simulink model "Three_phase"  (R2015a)
settings: Solver=ode45  StartTime=0.0  StopTime=10.0  RelTol=1e-3
undefined symbols (not defined in the file): Vdc
libraries: simulink x21
settings Model: Creator=Caner  LastModifiedBy=Caner

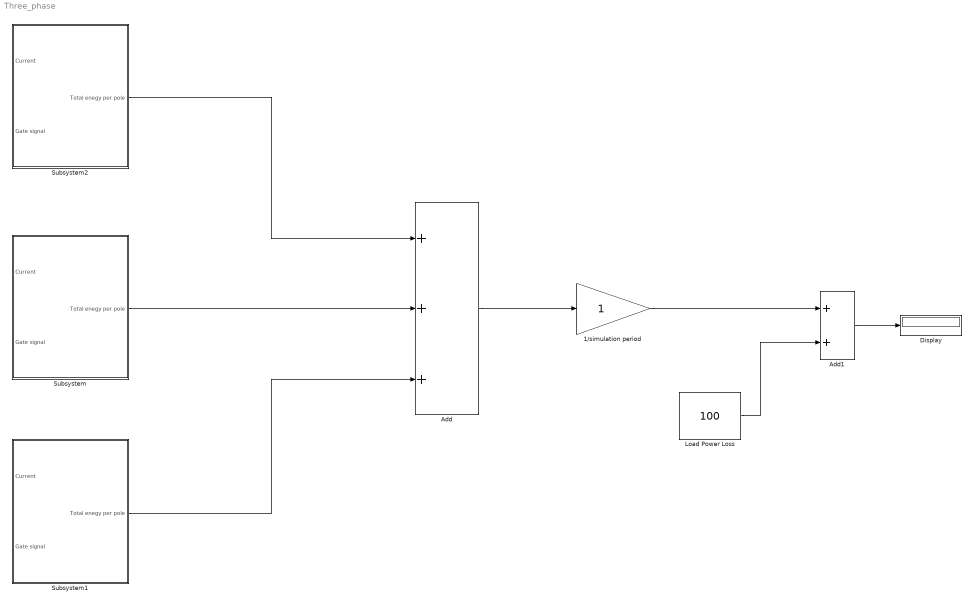
== system Three_phase ==
  1/simulation period : Gain
  Add : Sum  Inputs=+++
  Add1 : Sum
  Display : Display
  Load Power Loss : Constant  Value=100
  Subsystem : Subsystem
  Subsystem1 : Subsystem
  Subsystem2 : Subsystem
  wires:
  Subsystem2/1(Total enegy per pole) -> Add/1
  Subsystem/1(Total enegy per pole) -> Add/2
  Subsystem1/1(Total enegy per pole) -> Add/3
  Add/1 -> 1/simulation period/1
  1/simulation period/1 -> Add1/1
  Load Power Loss/1 -> Add1/2
  Add1/1 -> Display/1

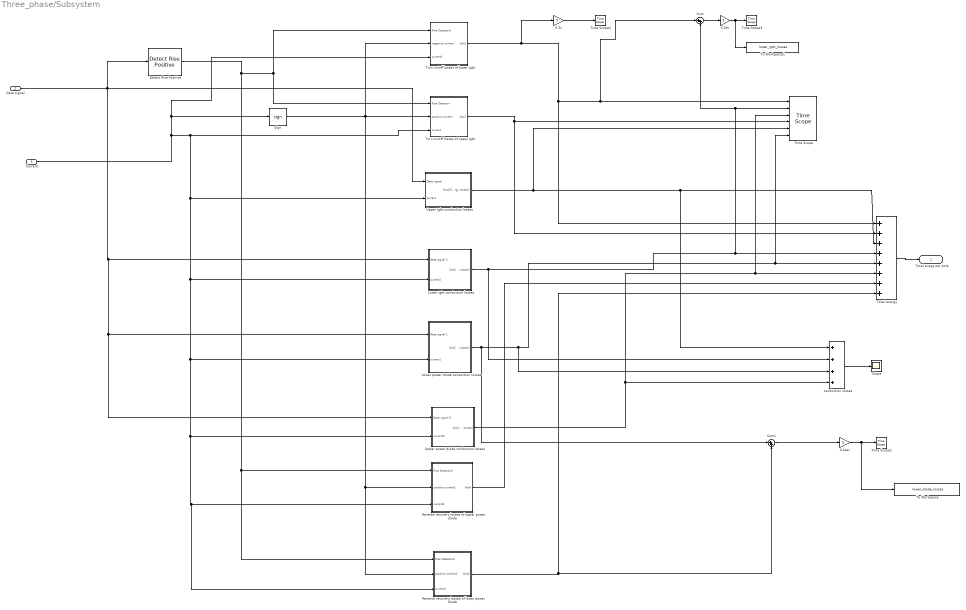
== system Three_phase/Subsystem ==
  Current : Inport
  "Gate signal " : Inport  Port=2
  0.2s : Gain  Gain=5
  0.2sec : Gain  Gain=5
  "0.2sn " : Gain  Gain=5
  Detect Rise Positive : simulink/Logic and Bit Operations/Detect Rise Positive  vinit=0  InputProcessing=Inherited  OutDataTypeStr=boolean
  Lower igbt conduction losses : Subsystem
  Lower power diode conduction losses : Subsystem
  "Reverse recovery losses of lower power diode " : Subsystem
  "Reverse recovery losses of upper power diode " : Subsystem
  Scope : Scope
      settings: SaveName=ScopeData3
  Sign : Signum
  Sum : Sum  Inputs=|++
  Sum1 : Sum  Inputs=|++
  Time Scope : TimeScope  DefaultConfigurationName=spbscopes.TimeScopeBlockCfg  NumInputPorts=6
  Time Scope1 : TimeScope  DefaultConfigurationName=spbscopes.TimeScopeBlockCfg
  Time Scope2 : TimeScope  DefaultConfigurationName=spbscopes.TimeScopeBlockCfg
  Time Scope3 : TimeScope  DefaultConfigurationName=spbscopes.TimeScopeBlockCfg
  To Workspace : ToWorkspace  VariableName=lower_diode_losses  SaveFormat=Timeseries  SampleTime=-1
  To Workspace1 : ToWorkspace  VariableName=lower_igbt_losses  SaveFormat=Timeseries  SampleTime=-1
  "Total energy " : Sum  Inputs=++++++++
  "Turn on/off losses of lower igbt " : Subsystem
  "Turn on/off losses of upper igbt " : Subsystem
  Upper igbt conduction losses : Subsystem
  Upper power diode conduction losses : Subsystem
  conduction losses : Sum  Inputs=++++
  Total enegy per pole : Outport
  wires:
  Current/1 -> Sign/1, "Turn on/off losses of lower igbt "/3(current1), "Turn on/off losses of upper igbt "/3(current), Upper igbt conduction losses/2(current), Lower igbt conduction losses/2(current2), Lower power diode conduction losses/2(current1), Upper power diode conduction losses/2(current3), "Reverse recovery losses of upper power diode "/3(current3), "Reverse recovery losses of lower power diode "/3(current2)
  Upper igbt conduction losses/1(Out1(Energy losses)) -> "Total energy "/3, conduction losses/1, Time Scope/5
  "Gate signal "/1 -> Detect Rise Positive/1, Upper igbt conduction losses/1("Gate signal "), Lower igbt conduction losses/1(Gate signal 2), Lower power diode conduction losses/1(Gate signal 1), Upper power diode conduction losses/1(Gate signal 3)
  Lower igbt conduction losses/1(Out3 (Energy losses)) -> "Total energy "/4, Sum/2, Time Scope/2, conduction losses/2
  "0.2sn "/1 -> Time Scope3/1, To Workspace1/1
  Detect Rise Positive/1 -> "Turn on/off losses of lower igbt "/1(Rise Detector1), "Turn on/off losses of upper igbt "/1(Rise Detector), "Reverse recovery losses of upper power diode "/1(Rise Detector3), "Reverse recovery losses of lower power diode "/1(Rise Detector2)
  Sum/1 -> "0.2sn "/1
  Upper power diode conduction losses/1(Out4 (Energy losses)) -> "Total energy "/6, Time Scope/3, conduction losses/4
  "Total energy "/1 -> Total enegy per pole/1
  0.2sec/1 -> Time Scope1/1, To Workspace/1
  Sum1/1 -> 0.2sec/1
  "Reverse recovery losses of upper power diode "/1(Out4) -> "Total energy "/7
  "Turn on/off losses of upper igbt "/1(Out1) -> Time Scope/4, "Total energy "/2
  conduction losses/1 -> Scope/1
  Sign/1 -> "Turn on/off losses of upper igbt "/2(positive current), "Turn on/off losses of lower igbt "/2(negative current), "Reverse recovery losses of lower power diode "/2(positive current1), "Reverse recovery losses of upper power diode "/2(positive current2)
  Lower power diode conduction losses/1(Out2 (Energy losses)) -> "Total energy "/5, Time Scope/6, conduction losses/3, Sum1/1
  0.2s/1 -> Time Scope2/1
  "Reverse recovery losses of lower power diode "/1(Out3) -> "Total energy "/8, Sum1/2
  "Turn on/off losses of lower igbt "/1(Out2) -> "Total energy "/1, Time Scope/1, Sum/1, 0.2s/1

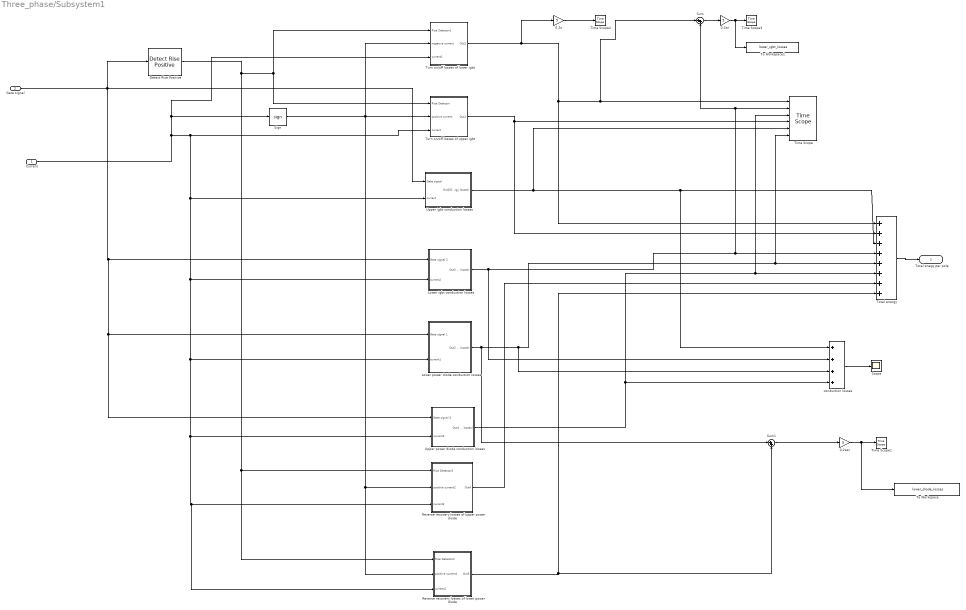
== system Three_phase/Subsystem1 ==
  Current : Inport
  "Gate signal " : Inport  Port=2
  0.2s : Gain  Gain=5
  0.2sec : Gain  Gain=5
  "0.2sn " : Gain  Gain=5
  Detect Rise Positive : simulink/Logic and Bit Operations/Detect Rise Positive  vinit=0  InputProcessing=Inherited  OutDataTypeStr=boolean
  Lower igbt conduction losses : Subsystem
  Lower power diode conduction losses : Subsystem
  "Reverse recovery losses of lower power diode " : Subsystem
  "Reverse recovery losses of upper power diode " : Subsystem
  Scope : Scope
      settings: SaveName=ScopeData3
  Sign : Signum
  Sum : Sum  Inputs=|++
  Sum1 : Sum  Inputs=|++
  Time Scope : TimeScope  DefaultConfigurationName=spbscopes.TimeScopeBlockCfg  NumInputPorts=6
  Time Scope1 : TimeScope  DefaultConfigurationName=spbscopes.TimeScopeBlockCfg
  Time Scope2 : TimeScope  DefaultConfigurationName=spbscopes.TimeScopeBlockCfg
  Time Scope3 : TimeScope  DefaultConfigurationName=spbscopes.TimeScopeBlockCfg
  To Workspace : ToWorkspace  VariableName=lower_diode_losses  SaveFormat=Timeseries  SampleTime=-1
  To Workspace1 : ToWorkspace  VariableName=lower_igbt_losses  SaveFormat=Timeseries  SampleTime=-1
  "Total energy " : Sum  Inputs=++++++++
  "Turn on/off losses of lower igbt " : Subsystem
  "Turn on/off losses of upper igbt " : Subsystem
  Upper igbt conduction losses : Subsystem
  Upper power diode conduction losses : Subsystem
  conduction losses : Sum  Inputs=++++
  Total enegy per pole : Outport
  wires:
  Current/1 -> Sign/1, "Turn on/off losses of lower igbt "/3(current1), "Turn on/off losses of upper igbt "/3(current), Upper igbt conduction losses/2(current), Lower igbt conduction losses/2(current2), Lower power diode conduction losses/2(current1), Upper power diode conduction losses/2(current3), "Reverse recovery losses of upper power diode "/3(current3), "Reverse recovery losses of lower power diode "/3(current2)
  Upper igbt conduction losses/1(Out1(Energy losses)) -> "Total energy "/3, conduction losses/1, Time Scope/5
  "Gate signal "/1 -> Detect Rise Positive/1, Upper igbt conduction losses/1("Gate signal "), Lower igbt conduction losses/1(Gate signal 2), Lower power diode conduction losses/1(Gate signal 1), Upper power diode conduction losses/1(Gate signal 3)
  Lower igbt conduction losses/1(Out3 (Energy losses)) -> "Total energy "/4, Sum/2, Time Scope/2, conduction losses/2
  "0.2sn "/1 -> Time Scope3/1, To Workspace1/1
  Detect Rise Positive/1 -> "Turn on/off losses of lower igbt "/1(Rise Detector1), "Turn on/off losses of upper igbt "/1(Rise Detector), "Reverse recovery losses of upper power diode "/1(Rise Detector3), "Reverse recovery losses of lower power diode "/1(Rise Detector2)
  Sum/1 -> "0.2sn "/1
  Upper power diode conduction losses/1(Out4 (Energy losses)) -> "Total energy "/6, Time Scope/3, conduction losses/4
  "Total energy "/1 -> Total enegy per pole/1
  0.2sec/1 -> Time Scope1/1, To Workspace/1
  Sum1/1 -> 0.2sec/1
  "Reverse recovery losses of upper power diode "/1(Out4) -> "Total energy "/7
  "Turn on/off losses of upper igbt "/1(Out1) -> Time Scope/4, "Total energy "/2
  conduction losses/1 -> Scope/1
  Sign/1 -> "Turn on/off losses of upper igbt "/2(positive current), "Turn on/off losses of lower igbt "/2(negative current), "Reverse recovery losses of lower power diode "/2(positive current1), "Reverse recovery losses of upper power diode "/2(positive current2)
  Lower power diode conduction losses/1(Out2 (Energy losses)) -> "Total energy "/5, Time Scope/6, conduction losses/3, Sum1/1
  0.2s/1 -> Time Scope2/1
  "Reverse recovery losses of lower power diode "/1(Out3) -> "Total energy "/8, Sum1/2
  "Turn on/off losses of lower igbt "/1(Out2) -> "Total energy "/1, Time Scope/1, Sum/1, 0.2s/1

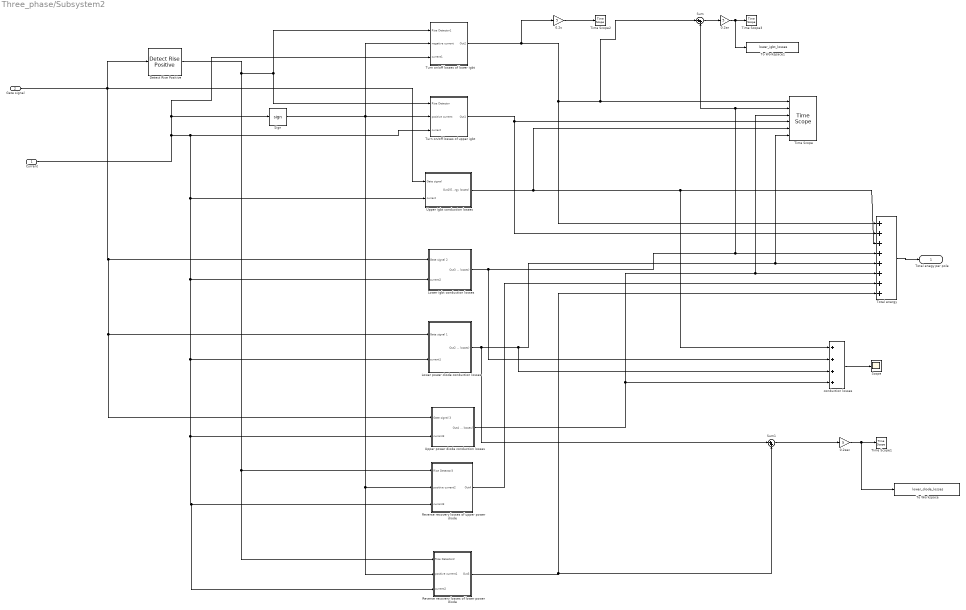
== system Three_phase/Subsystem2 ==
  Current : Inport
  "Gate signal " : Inport  Port=2
  0.2s : Gain  Gain=5
  0.2sec : Gain  Gain=5
  "0.2sn " : Gain  Gain=5
  Detect Rise Positive : simulink/Logic and Bit Operations/Detect Rise Positive  vinit=0  InputProcessing=Inherited  OutDataTypeStr=boolean
  Lower igbt conduction losses : Subsystem
  Lower power diode conduction losses : Subsystem
  "Reverse recovery losses of lower power diode " : Subsystem
  "Reverse recovery losses of upper power diode " : Subsystem
  Scope : Scope
      settings: SaveName=ScopeData3
  Sign : Signum
  Sum : Sum  Inputs=|++
  Sum1 : Sum  Inputs=|++
  Time Scope : TimeScope  DefaultConfigurationName=spbscopes.TimeScopeBlockCfg  NumInputPorts=6
  Time Scope1 : TimeScope  DefaultConfigurationName=spbscopes.TimeScopeBlockCfg
  Time Scope2 : TimeScope  DefaultConfigurationName=spbscopes.TimeScopeBlockCfg
  Time Scope3 : TimeScope  DefaultConfigurationName=spbscopes.TimeScopeBlockCfg
  To Workspace : ToWorkspace  VariableName=lower_diode_losses  SaveFormat=Timeseries  SampleTime=-1
  To Workspace1 : ToWorkspace  VariableName=lower_igbt_losses  SaveFormat=Timeseries  SampleTime=-1
  "Total energy " : Sum  Inputs=++++++++
  "Turn on/off losses of lower igbt " : Subsystem
  "Turn on/off losses of upper igbt " : Subsystem
  Upper igbt conduction losses : Subsystem
  Upper power diode conduction losses : Subsystem
  conduction losses : Sum  Inputs=++++
  Total enegy per pole : Outport
  wires:
  Current/1 -> Sign/1, "Turn on/off losses of lower igbt "/3(current1), "Turn on/off losses of upper igbt "/3(current), Upper igbt conduction losses/2(current), Lower igbt conduction losses/2(current2), Lower power diode conduction losses/2(current1), Upper power diode conduction losses/2(current3), "Reverse recovery losses of upper power diode "/3(current3), "Reverse recovery losses of lower power diode "/3(current2)
  Upper igbt conduction losses/1(Out1(Energy losses)) -> "Total energy "/3, conduction losses/1, Time Scope/5
  "Gate signal "/1 -> Detect Rise Positive/1, Upper igbt conduction losses/1("Gate signal "), Lower igbt conduction losses/1(Gate signal 2), Lower power diode conduction losses/1(Gate signal 1), Upper power diode conduction losses/1(Gate signal 3)
  Lower igbt conduction losses/1(Out3 (Energy losses)) -> "Total energy "/4, Sum/2, Time Scope/2, conduction losses/2
  "0.2sn "/1 -> Time Scope3/1, To Workspace1/1
  Detect Rise Positive/1 -> "Turn on/off losses of lower igbt "/1(Rise Detector1), "Turn on/off losses of upper igbt "/1(Rise Detector), "Reverse recovery losses of upper power diode "/1(Rise Detector3), "Reverse recovery losses of lower power diode "/1(Rise Detector2)
  Sum/1 -> "0.2sn "/1
  Upper power diode conduction losses/1(Out4 (Energy losses)) -> "Total energy "/6, Time Scope/3, conduction losses/4
  "Total energy "/1 -> Total enegy per pole/1
  0.2sec/1 -> Time Scope1/1, To Workspace/1
  Sum1/1 -> 0.2sec/1
  "Reverse recovery losses of upper power diode "/1(Out4) -> "Total energy "/7
  "Turn on/off losses of upper igbt "/1(Out1) -> Time Scope/4, "Total energy "/2
  conduction losses/1 -> Scope/1
  Sign/1 -> "Turn on/off losses of upper igbt "/2(positive current), "Turn on/off losses of lower igbt "/2(negative current), "Reverse recovery losses of lower power diode "/2(positive current1), "Reverse recovery losses of upper power diode "/2(positive current2)
  Lower power diode conduction losses/1(Out2 (Energy losses)) -> "Total energy "/5, Time Scope/6, conduction losses/3, Sum1/1
  0.2s/1 -> Time Scope2/1
  "Reverse recovery losses of lower power diode "/1(Out3) -> "Total energy "/8, Sum1/2
  "Turn on/off losses of lower igbt "/1(Out2) -> "Total energy "/1, Time Scope/1, Sum/1, 0.2s/1

== system Three_phase/Subsystem/Lower igbt conduction losses ==
  note: Lower igbt conduction losses
  Gate signal 2 : Inport
  current2 : Inport  Port=2
  Abs : Abs
  Compare To Zero3 : simulink/Logic and Bit Operations/Compare To Zero  relop=<  OutDataTypeStr=boolean
  Compare To Zero4 : simulink/Logic and Bit Operations/Compare To Zero  relop===  OutDataTypeStr=boolean
  Integrator2 : Integrator
  Logical Operator2 : Logic  AllPortsSameDT=off  OutDataTypeStr=boolean
  Product2 : Product
  Vec1 : Gain  Gain=1.8
  Out3 (Energy losses) : Outport
  wires:
  Gate signal 2/1 -> Compare To Zero4/1
  Compare To Zero3/1 -> Logical Operator2/2
  current2/1 -> Abs/1, Compare To Zero3/1
  Vec1/1 -> Integrator2/1
  Abs/1 -> Product2/2
  Compare To Zero4/1 -> Logical Operator2/1
  Product2/1 -> Vec1/1
  Integrator2/1 -> Out3 (Energy losses)/1
  Logical Operator2/1 -> Product2/1

== system Three_phase/Subsystem/Lower power diode conduction losses ==
  note: Lower power diode conduction losses
  Gate signal 1 : Inport
  current1 : Inport  Port=2
  Compare To Zero1 : simulink/Logic and Bit Operations/Compare To Zero  relop=>  OutDataTypeStr=boolean
  Compare To Zero2 : simulink/Logic and Bit Operations/Compare To Zero  relop===  OutDataTypeStr=boolean
  Integrator1 : Integrator
  Logical Operator1 : Logic  AllPortsSameDT=off  OutDataTypeStr=boolean
  Product1 : Product
  Vec : Gain  Gain=1.8
  Out2 (Energy losses) : Outport
  wires:
  Compare To Zero1/1 -> Logical Operator1/2
  Logical Operator1/1 -> Product1/1
  Gate signal 1/1 -> Compare To Zero2/1
  current1/1 -> Product1/2, Compare To Zero1/1
  Compare To Zero2/1 -> Logical Operator1/1
  Vec/1 -> Integrator1/1
  Integrator1/1 -> Out2 (Energy losses)/1
  Product1/1 -> Vec/1

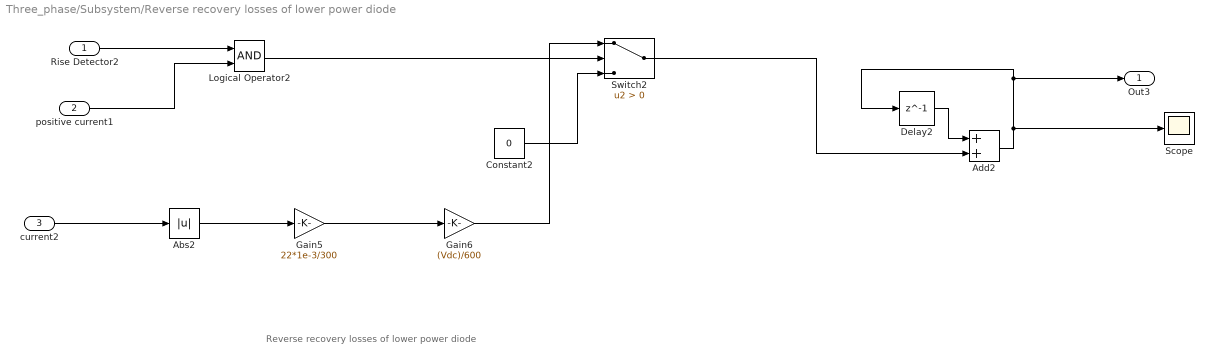
== system Three_phase/Subsystem/Reverse recovery losses of lower power diode  ==
  note: Reverse recovery losses of lower power diode
  Rise Detector2 : Inport
  positive current1 : Inport  Port=2
  current2 : Inport  Port=3
  Abs2 : Abs
  Add2 : Sum
  Constant2 : Constant  Value=0
  Delay2 : Delay  DelayLength=1  InitialCondition=0
  Gain5 : Gain  Gain=22*1e-3/300
  Gain6 : Gain  Gain=(Vdc)/600
  Logical Operator2 : Logic  AllPortsSameDT=off  OutDataTypeStr=boolean
  Scope : Scope
  Switch2 : Switch  Criteria=u2 > Threshold
  Out3 : Outport
  wires:
  Gain5/1 -> Gain6/1
  Constant2/1 -> Switch2/3
  positive current1/1 -> Logical Operator2/2
  Add2/1 -> Scope/1, Out3/1, Delay2/1
  current2/1 -> Abs2/1
  Logical Operator2/1 -> Switch2/2
  Gain6/1 -> Switch2/1
  Rise Detector2/1 -> Logical Operator2/1
  Switch2/1 -> Add2/2
  Delay2/1 -> Add2/1
  Abs2/1 -> Gain5/1

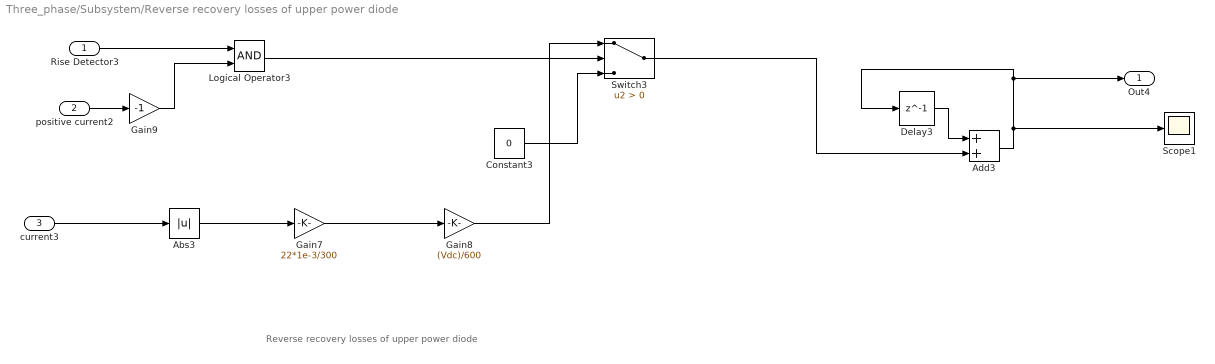
== system Three_phase/Subsystem/Reverse recovery losses of upper power diode  ==
  note: Reverse recovery losses of upper power diode
  Rise Detector3 : Inport
  positive current2 : Inport  Port=2
  current3 : Inport  Port=3
  Abs3 : Abs
  Add3 : Sum
  Constant3 : Constant  Value=0
  Delay3 : Delay  DelayLength=1  InitialCondition=0
  Gain7 : Gain  Gain=22*1e-3/300
  Gain8 : Gain  Gain=(Vdc)/600
  Gain9 : Gain  Gain=-1
  Logical Operator3 : Logic  AllPortsSameDT=off  OutDataTypeStr=boolean
  Scope1 : Scope
  Switch3 : Switch  Criteria=u2 > Threshold
  Out4 : Outport
  wires:
  Abs3/1 -> Gain7/1
  Gain7/1 -> Gain8/1
  Gain8/1 -> Switch3/1
  Rise Detector3/1 -> Logical Operator3/1
  positive current2/1 -> Gain9/1
  Logical Operator3/1 -> Switch3/2
  current3/1 -> Abs3/1
  Add3/1 -> Scope1/1, Out4/1, Delay3/1
  Delay3/1 -> Add3/1
  Constant3/1 -> Switch3/3
  Gain9/1 -> Logical Operator3/2
  Switch3/1 -> Add3/2

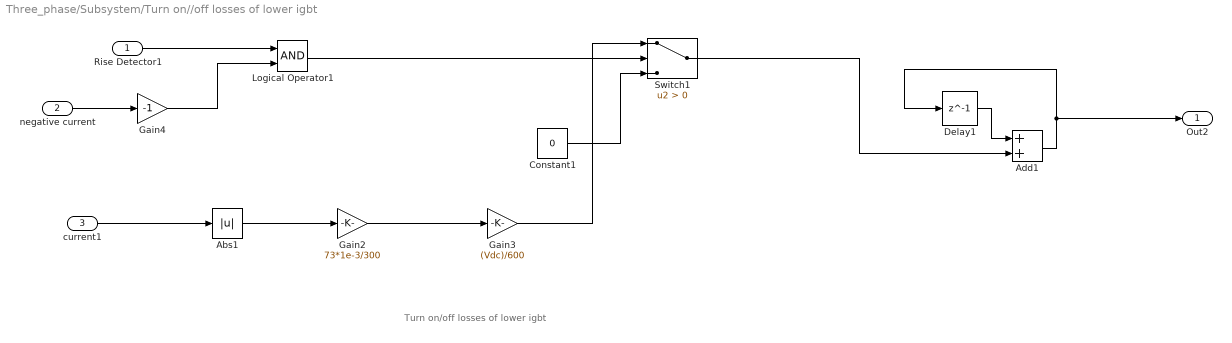
== system Three_phase/Subsystem/Turn on//off losses of lower igbt  ==
  note: Turn on/off losses of lower igbt
  Rise Detector1 : Inport
  negative current : Inport  Port=2
  current1 : Inport  Port=3
  Abs1 : Abs
  Add1 : Sum
  Constant1 : Constant  Value=0
  Delay1 : Delay  DelayLength=1  InitialCondition=0
  Gain2 : Gain  Gain=73*1e-3/300
  Gain3 : Gain  Gain=(Vdc)/600
  Gain4 : Gain  Gain=-1
  Logical Operator1 : Logic  AllPortsSameDT=off  OutDataTypeStr=boolean
  Switch1 : Switch  Criteria=u2 > Threshold
  Out2 : Outport
  wires:
  Delay1/1 -> Add1/1
  current1/1 -> Abs1/1
  Gain3/1 -> Switch1/1
  Constant1/1 -> Switch1/3
  Gain4/1 -> Logical Operator1/2
  Logical Operator1/1 -> Switch1/2
  negative current/1 -> Gain4/1
  Rise Detector1/1 -> Logical Operator1/1
  Abs1/1 -> Gain2/1
  Add1/1 -> Out2/1, Delay1/1
  Gain2/1 -> Gain3/1
  Switch1/1 -> Add1/2

== system Three_phase/Subsystem/Turn on//off losses of upper igbt  ==
  note: Turn on/off losses of upper igbt
  Rise Detector : Inport
  positive current : Inport  Port=2
  current : Inport  Port=3
  Abs : Abs
  Add : Sum
  Constant : Constant  Value=0
  Delay : Delay  DelayLength=1  InitialCondition=0
  Gain : Gain  Gain=73*1e-3/300
  Gain1 : Gain  Gain=(Vdc)/600
  Logical Operator : Logic  AllPortsSameDT=off  OutDataTypeStr=boolean
  Switch : Switch  Criteria=u2 > Threshold
  Out1 : Outport
  wires:
  Add/1 -> Out1/1, Delay/1
  Logical Operator/1 -> Switch/2
  current/1 -> Abs/1
  Abs/1 -> Gain/1
  Rise Detector/1 -> Logical Operator/1
  positive current/1 -> Logical Operator/2
  Gain/1 -> Gain1/1
  Gain1/1 -> Switch/1
  Constant/1 -> Switch/3
  Delay/1 -> Add/1
  Switch/1 -> Add/2

== system Three_phase/Subsystem/Upper igbt conduction losses ==
  note: Upper igbt conduction losses
  "Gate signal " : Inport
  current : Inport  Port=2
  Compare To Zero : simulink/Logic and Bit Operations/Compare To Zero  relop=>  OutDataTypeStr=boolean
  Integrator : Integrator
  Logical Operator : Logic  AllPortsSameDT=off  OutDataTypeStr=boolean
  Product : Product
  Vce : Gain  Gain=1.8
  Out1(Energy losses) : Outport
  wires:
  Compare To Zero/1 -> Logical Operator/2
  current/1 -> Product/2, Compare To Zero/1
  Integrator/1 -> Out1(Energy losses)/1
  "Gate signal "/1 -> Logical Operator/1
  Product/1 -> Vce/1
  Vce/1 -> Integrator/1
  Logical Operator/1 -> Product/1

== system Three_phase/Subsystem/Upper power diode conduction losses ==
  note: Upper power diode conduction losses
  Gate signal 3 : Inport
  current3 : Inport  Port=2
  Abs1 : Abs
  Compare To Zero5 : simulink/Logic and Bit Operations/Compare To Zero  relop=<  OutDataTypeStr=boolean
  Integrator3 : Integrator
  Logical Operator3 : Logic  AllPortsSameDT=off  OutDataTypeStr=boolean
  Product3 : Product
  Vec2 : Gain  Gain=1.8
  Out4 (Energy losses) : Outport
  wires:
  Product3/1 -> Vec2/1
  current3/1 -> Abs1/1, Compare To Zero5/1
  Abs1/1 -> Product3/2
  Compare To Zero5/1 -> Logical Operator3/2
  Gate signal 3/1 -> Logical Operator3/1
  Vec2/1 -> Integrator3/1
  Integrator3/1 -> Out4 (Energy losses)/1
  Logical Operator3/1 -> Product3/1

== system Three_phase/Subsystem1/Lower igbt conduction losses ==
  note: Lower igbt conduction losses
  Gate signal 2 : Inport
  current2 : Inport  Port=2
  Abs : Abs
  Compare To Zero3 : simulink/Logic and Bit Operations/Compare To Zero  relop=<  OutDataTypeStr=boolean
  Compare To Zero4 : simulink/Logic and Bit Operations/Compare To Zero  relop===  OutDataTypeStr=boolean
  Integrator2 : Integrator
  Logical Operator2 : Logic  AllPortsSameDT=off  OutDataTypeStr=boolean
  Product2 : Product
  Vec1 : Gain  Gain=1.8
  Out3 (Energy losses) : Outport
  wires:
  Gate signal 2/1 -> Compare To Zero4/1
  Compare To Zero3/1 -> Logical Operator2/2
  current2/1 -> Abs/1, Compare To Zero3/1
  Vec1/1 -> Integrator2/1
  Abs/1 -> Product2/2
  Compare To Zero4/1 -> Logical Operator2/1
  Product2/1 -> Vec1/1
  Integrator2/1 -> Out3 (Energy losses)/1
  Logical Operator2/1 -> Product2/1

== system Three_phase/Subsystem1/Lower power diode conduction losses ==
  note: Lower power diode conduction losses
  Gate signal 1 : Inport
  current1 : Inport  Port=2
  Compare To Zero1 : simulink/Logic and Bit Operations/Compare To Zero  relop=>  OutDataTypeStr=boolean
  Compare To Zero2 : simulink/Logic and Bit Operations/Compare To Zero  relop===  OutDataTypeStr=boolean
  Integrator1 : Integrator
  Logical Operator1 : Logic  AllPortsSameDT=off  OutDataTypeStr=boolean
  Product1 : Product
  Vec : Gain  Gain=1.8
  Out2 (Energy losses) : Outport
  wires:
  Compare To Zero1/1 -> Logical Operator1/2
  Logical Operator1/1 -> Product1/1
  Gate signal 1/1 -> Compare To Zero2/1
  current1/1 -> Product1/2, Compare To Zero1/1
  Compare To Zero2/1 -> Logical Operator1/1
  Vec/1 -> Integrator1/1
  Integrator1/1 -> Out2 (Energy losses)/1
  Product1/1 -> Vec/1

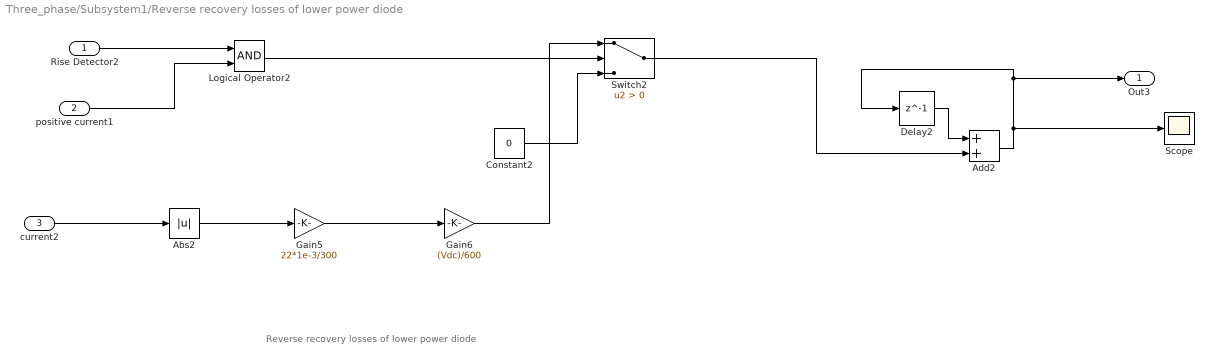
== system Three_phase/Subsystem1/Reverse recovery losses of lower power diode  ==
  note: Reverse recovery losses of lower power diode
  Rise Detector2 : Inport
  positive current1 : Inport  Port=2
  current2 : Inport  Port=3
  Abs2 : Abs
  Add2 : Sum
  Constant2 : Constant  Value=0
  Delay2 : Delay  DelayLength=1  InitialCondition=0
  Gain5 : Gain  Gain=22*1e-3/300
  Gain6 : Gain  Gain=(Vdc)/600
  Logical Operator2 : Logic  AllPortsSameDT=off  OutDataTypeStr=boolean
  Scope : Scope
  Switch2 : Switch  Criteria=u2 > Threshold
  Out3 : Outport
  wires:
  Gain5/1 -> Gain6/1
  Constant2/1 -> Switch2/3
  positive current1/1 -> Logical Operator2/2
  Add2/1 -> Scope/1, Out3/1, Delay2/1
  current2/1 -> Abs2/1
  Logical Operator2/1 -> Switch2/2
  Gain6/1 -> Switch2/1
  Rise Detector2/1 -> Logical Operator2/1
  Switch2/1 -> Add2/2
  Delay2/1 -> Add2/1
  Abs2/1 -> Gain5/1

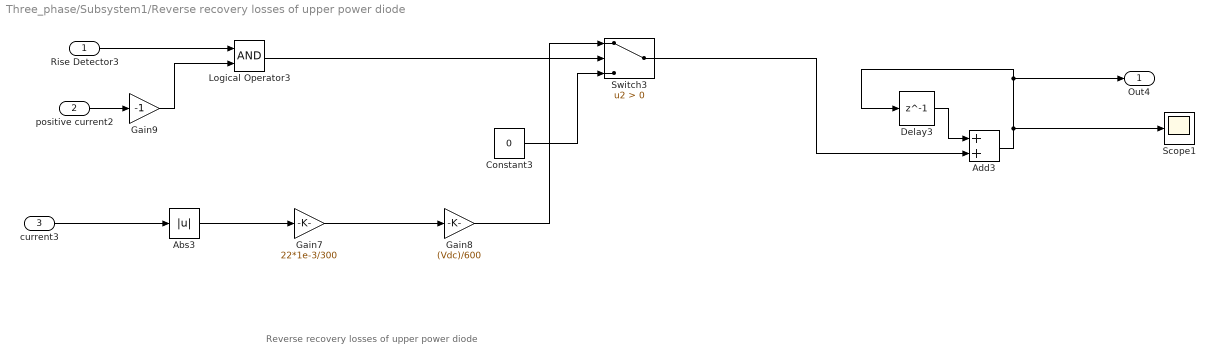
== system Three_phase/Subsystem1/Reverse recovery losses of upper power diode  ==
  note: Reverse recovery losses of upper power diode
  Rise Detector3 : Inport
  positive current2 : Inport  Port=2
  current3 : Inport  Port=3
  Abs3 : Abs
  Add3 : Sum
  Constant3 : Constant  Value=0
  Delay3 : Delay  DelayLength=1  InitialCondition=0
  Gain7 : Gain  Gain=22*1e-3/300
  Gain8 : Gain  Gain=(Vdc)/600
  Gain9 : Gain  Gain=-1
  Logical Operator3 : Logic  AllPortsSameDT=off  OutDataTypeStr=boolean
  Scope1 : Scope
  Switch3 : Switch  Criteria=u2 > Threshold
  Out4 : Outport
  wires:
  Abs3/1 -> Gain7/1
  Gain7/1 -> Gain8/1
  Gain8/1 -> Switch3/1
  Rise Detector3/1 -> Logical Operator3/1
  positive current2/1 -> Gain9/1
  Logical Operator3/1 -> Switch3/2
  current3/1 -> Abs3/1
  Add3/1 -> Scope1/1, Out4/1, Delay3/1
  Delay3/1 -> Add3/1
  Constant3/1 -> Switch3/3
  Gain9/1 -> Logical Operator3/2
  Switch3/1 -> Add3/2

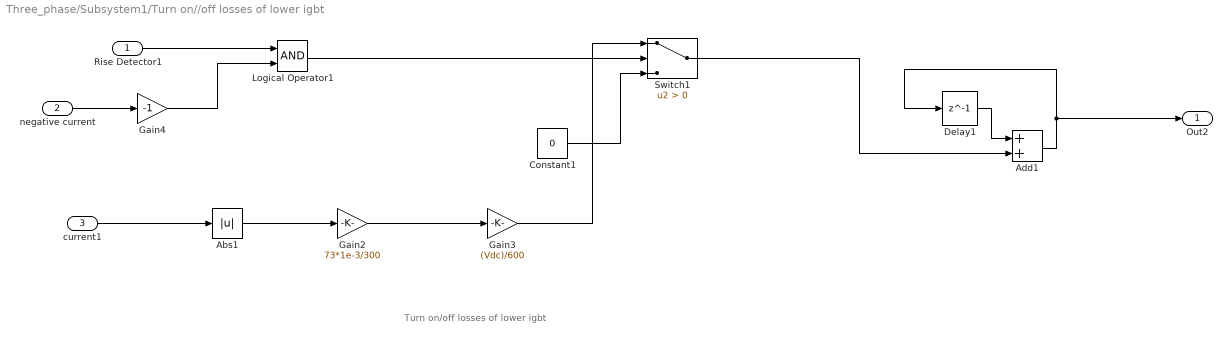
== system Three_phase/Subsystem1/Turn on//off losses of lower igbt  ==
  note: Turn on/off losses of lower igbt
  Rise Detector1 : Inport
  negative current : Inport  Port=2
  current1 : Inport  Port=3
  Abs1 : Abs
  Add1 : Sum
  Constant1 : Constant  Value=0
  Delay1 : Delay  DelayLength=1  InitialCondition=0
  Gain2 : Gain  Gain=73*1e-3/300
  Gain3 : Gain  Gain=(Vdc)/600
  Gain4 : Gain  Gain=-1
  Logical Operator1 : Logic  AllPortsSameDT=off  OutDataTypeStr=boolean
  Switch1 : Switch  Criteria=u2 > Threshold
  Out2 : Outport
  wires:
  Delay1/1 -> Add1/1
  current1/1 -> Abs1/1
  Gain3/1 -> Switch1/1
  Constant1/1 -> Switch1/3
  Gain4/1 -> Logical Operator1/2
  Logical Operator1/1 -> Switch1/2
  negative current/1 -> Gain4/1
  Rise Detector1/1 -> Logical Operator1/1
  Abs1/1 -> Gain2/1
  Add1/1 -> Out2/1, Delay1/1
  Gain2/1 -> Gain3/1
  Switch1/1 -> Add1/2

== system Three_phase/Subsystem1/Turn on//off losses of upper igbt  ==
  note: Turn on/off losses of upper igbt
  Rise Detector : Inport
  positive current : Inport  Port=2
  current : Inport  Port=3
  Abs : Abs
  Add : Sum
  Constant : Constant  Value=0
  Delay : Delay  DelayLength=1  InitialCondition=0
  Gain : Gain  Gain=73*1e-3/300
  Gain1 : Gain  Gain=(Vdc)/600
  Logical Operator : Logic  AllPortsSameDT=off  OutDataTypeStr=boolean
  Switch : Switch  Criteria=u2 > Threshold
  Out1 : Outport
  wires:
  Add/1 -> Out1/1, Delay/1
  Logical Operator/1 -> Switch/2
  current/1 -> Abs/1
  Abs/1 -> Gain/1
  Rise Detector/1 -> Logical Operator/1
  positive current/1 -> Logical Operator/2
  Gain/1 -> Gain1/1
  Gain1/1 -> Switch/1
  Constant/1 -> Switch/3
  Delay/1 -> Add/1
  Switch/1 -> Add/2

== system Three_phase/Subsystem1/Upper igbt conduction losses ==
  note: Upper igbt conduction losses
  "Gate signal " : Inport
  current : Inport  Port=2
  Compare To Zero : simulink/Logic and Bit Operations/Compare To Zero  relop=>  OutDataTypeStr=boolean
  Integrator : Integrator
  Logical Operator : Logic  AllPortsSameDT=off  OutDataTypeStr=boolean
  Product : Product
  Vce : Gain  Gain=1.8
  Out1(Energy losses) : Outport
  wires:
  Compare To Zero/1 -> Logical Operator/2
  current/1 -> Product/2, Compare To Zero/1
  Integrator/1 -> Out1(Energy losses)/1
  "Gate signal "/1 -> Logical Operator/1
  Product/1 -> Vce/1
  Vce/1 -> Integrator/1
  Logical Operator/1 -> Product/1

== system Three_phase/Subsystem1/Upper power diode conduction losses ==
  note: Upper power diode conduction losses
  Gate signal 3 : Inport
  current3 : Inport  Port=2
  Abs1 : Abs
  Compare To Zero5 : simulink/Logic and Bit Operations/Compare To Zero  relop=<  OutDataTypeStr=boolean
  Integrator3 : Integrator
  Logical Operator3 : Logic  AllPortsSameDT=off  OutDataTypeStr=boolean
  Product3 : Product
  Vec2 : Gain  Gain=1.8
  Out4 (Energy losses) : Outport
  wires:
  Product3/1 -> Vec2/1
  current3/1 -> Abs1/1, Compare To Zero5/1
  Abs1/1 -> Product3/2
  Compare To Zero5/1 -> Logical Operator3/2
  Gate signal 3/1 -> Logical Operator3/1
  Vec2/1 -> Integrator3/1
  Integrator3/1 -> Out4 (Energy losses)/1
  Logical Operator3/1 -> Product3/1

== system Three_phase/Subsystem2/Lower igbt conduction losses ==
  note: Lower igbt conduction losses
  Gate signal 2 : Inport
  current2 : Inport  Port=2
  Abs : Abs
  Compare To Zero3 : simulink/Logic and Bit Operations/Compare To Zero  relop=<  OutDataTypeStr=boolean
  Compare To Zero4 : simulink/Logic and Bit Operations/Compare To Zero  relop===  OutDataTypeStr=boolean
  Integrator2 : Integrator
  Logical Operator2 : Logic  AllPortsSameDT=off  OutDataTypeStr=boolean
  Product2 : Product
  Vec1 : Gain  Gain=1.8
  Out3 (Energy losses) : Outport
  wires:
  Gate signal 2/1 -> Compare To Zero4/1
  Compare To Zero3/1 -> Logical Operator2/2
  current2/1 -> Abs/1, Compare To Zero3/1
  Vec1/1 -> Integrator2/1
  Abs/1 -> Product2/2
  Compare To Zero4/1 -> Logical Operator2/1
  Product2/1 -> Vec1/1
  Integrator2/1 -> Out3 (Energy losses)/1
  Logical Operator2/1 -> Product2/1

== system Three_phase/Subsystem2/Lower power diode conduction losses ==
  note: Lower power diode conduction losses
  Gate signal 1 : Inport
  current1 : Inport  Port=2
  Compare To Zero1 : simulink/Logic and Bit Operations/Compare To Zero  relop=>  OutDataTypeStr=boolean
  Compare To Zero2 : simulink/Logic and Bit Operations/Compare To Zero  relop===  OutDataTypeStr=boolean
  Integrator1 : Integrator
  Logical Operator1 : Logic  AllPortsSameDT=off  OutDataTypeStr=boolean
  Product1 : Product
  Vec : Gain  Gain=1.8
  Out2 (Energy losses) : Outport
  wires:
  Compare To Zero1/1 -> Logical Operator1/2
  Logical Operator1/1 -> Product1/1
  Gate signal 1/1 -> Compare To Zero2/1
  current1/1 -> Product1/2, Compare To Zero1/1
  Compare To Zero2/1 -> Logical Operator1/1
  Vec/1 -> Integrator1/1
  Integrator1/1 -> Out2 (Energy losses)/1
  Product1/1 -> Vec/1

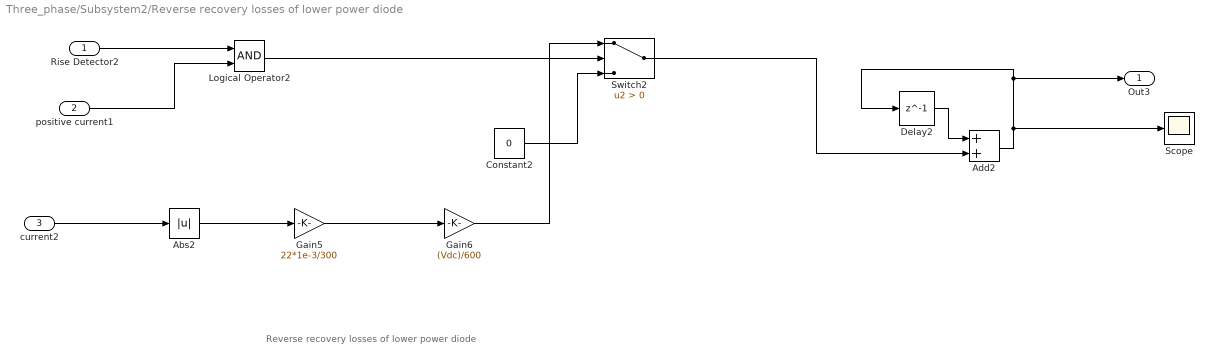
== system Three_phase/Subsystem2/Reverse recovery losses of lower power diode  ==
  note: Reverse recovery losses of lower power diode
  Rise Detector2 : Inport
  positive current1 : Inport  Port=2
  current2 : Inport  Port=3
  Abs2 : Abs
  Add2 : Sum
  Constant2 : Constant  Value=0
  Delay2 : Delay  DelayLength=1  InitialCondition=0
  Gain5 : Gain  Gain=22*1e-3/300
  Gain6 : Gain  Gain=(Vdc)/600
  Logical Operator2 : Logic  AllPortsSameDT=off  OutDataTypeStr=boolean
  Scope : Scope
  Switch2 : Switch  Criteria=u2 > Threshold
  Out3 : Outport
  wires:
  Gain5/1 -> Gain6/1
  Constant2/1 -> Switch2/3
  positive current1/1 -> Logical Operator2/2
  Add2/1 -> Scope/1, Out3/1, Delay2/1
  current2/1 -> Abs2/1
  Logical Operator2/1 -> Switch2/2
  Gain6/1 -> Switch2/1
  Rise Detector2/1 -> Logical Operator2/1
  Switch2/1 -> Add2/2
  Delay2/1 -> Add2/1
  Abs2/1 -> Gain5/1

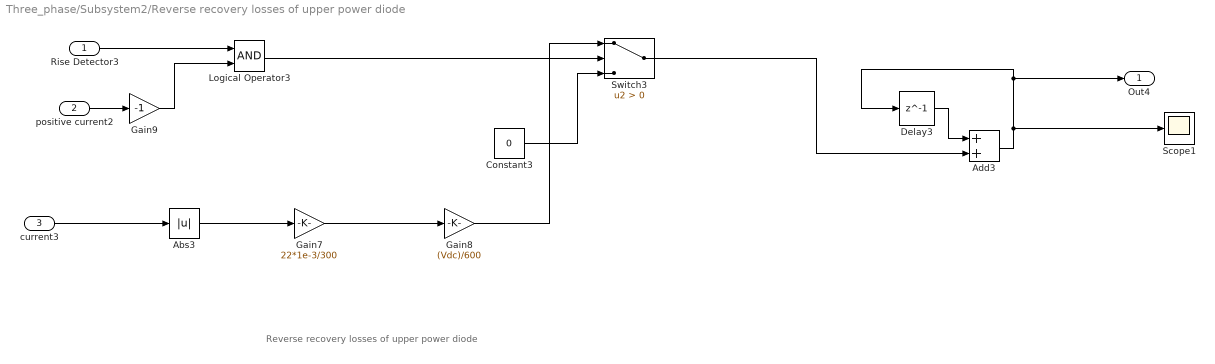
== system Three_phase/Subsystem2/Reverse recovery losses of upper power diode  ==
  note: Reverse recovery losses of upper power diode
  Rise Detector3 : Inport
  positive current2 : Inport  Port=2
  current3 : Inport  Port=3
  Abs3 : Abs
  Add3 : Sum
  Constant3 : Constant  Value=0
  Delay3 : Delay  DelayLength=1  InitialCondition=0
  Gain7 : Gain  Gain=22*1e-3/300
  Gain8 : Gain  Gain=(Vdc)/600
  Gain9 : Gain  Gain=-1
  Logical Operator3 : Logic  AllPortsSameDT=off  OutDataTypeStr=boolean
  Scope1 : Scope
  Switch3 : Switch  Criteria=u2 > Threshold
  Out4 : Outport
  wires:
  Abs3/1 -> Gain7/1
  Gain7/1 -> Gain8/1
  Gain8/1 -> Switch3/1
  Rise Detector3/1 -> Logical Operator3/1
  positive current2/1 -> Gain9/1
  Logical Operator3/1 -> Switch3/2
  current3/1 -> Abs3/1
  Add3/1 -> Scope1/1, Out4/1, Delay3/1
  Delay3/1 -> Add3/1
  Constant3/1 -> Switch3/3
  Gain9/1 -> Logical Operator3/2
  Switch3/1 -> Add3/2

== system Three_phase/Subsystem2/Turn on//off losses of lower igbt  ==
  note: Turn on/off losses of lower igbt
  Rise Detector1 : Inport
  negative current : Inport  Port=2
  current1 : Inport  Port=3
  Abs1 : Abs
  Add1 : Sum
  Constant1 : Constant  Value=0
  Delay1 : Delay  DelayLength=1  InitialCondition=0
  Gain2 : Gain  Gain=73*1e-3/300
  Gain3 : Gain  Gain=(Vdc)/600
  Gain4 : Gain  Gain=-1
  Logical Operator1 : Logic  AllPortsSameDT=off  OutDataTypeStr=boolean
  Switch1 : Switch  Criteria=u2 > Threshold
  Out2 : Outport
  wires:
  Delay1/1 -> Add1/1
  current1/1 -> Abs1/1
  Gain3/1 -> Switch1/1
  Constant1/1 -> Switch1/3
  Gain4/1 -> Logical Operator1/2
  Logical Operator1/1 -> Switch1/2
  negative current/1 -> Gain4/1
  Rise Detector1/1 -> Logical Operator1/1
  Abs1/1 -> Gain2/1
  Add1/1 -> Out2/1, Delay1/1
  Gain2/1 -> Gain3/1
  Switch1/1 -> Add1/2

== system Three_phase/Subsystem2/Turn on//off losses of upper igbt  ==
  note: Turn on/off losses of upper igbt
  Rise Detector : Inport
  positive current : Inport  Port=2
  current : Inport  Port=3
  Abs : Abs
  Add : Sum
  Constant : Constant  Value=0
  Delay : Delay  DelayLength=1  InitialCondition=0
  Gain : Gain  Gain=73*1e-3/300
  Gain1 : Gain  Gain=(Vdc)/600
  Logical Operator : Logic  AllPortsSameDT=off  OutDataTypeStr=boolean
  Switch : Switch  Criteria=u2 > Threshold
  Out1 : Outport
  wires:
  Add/1 -> Out1/1, Delay/1
  Logical Operator/1 -> Switch/2
  current/1 -> Abs/1
  Abs/1 -> Gain/1
  Rise Detector/1 -> Logical Operator/1
  positive current/1 -> Logical Operator/2
  Gain/1 -> Gain1/1
  Gain1/1 -> Switch/1
  Constant/1 -> Switch/3
  Delay/1 -> Add/1
  Switch/1 -> Add/2

== system Three_phase/Subsystem2/Upper igbt conduction losses ==
  note: Upper igbt conduction losses
  "Gate signal " : Inport
  current : Inport  Port=2
  Compare To Zero : simulink/Logic and Bit Operations/Compare To Zero  relop=>  OutDataTypeStr=boolean
  Integrator : Integrator
  Logical Operator : Logic  AllPortsSameDT=off  OutDataTypeStr=boolean
  Product : Product
  Vce : Gain  Gain=1.8
  Out1(Energy losses) : Outport
  wires:
  Compare To Zero/1 -> Logical Operator/2
  current/1 -> Product/2, Compare To Zero/1
  Integrator/1 -> Out1(Energy losses)/1
  "Gate signal "/1 -> Logical Operator/1
  Product/1 -> Vce/1
  Vce/1 -> Integrator/1
  Logical Operator/1 -> Product/1

== system Three_phase/Subsystem2/Upper power diode conduction losses ==
  note: Upper power diode conduction losses
  Gate signal 3 : Inport
  current3 : Inport  Port=2
  Abs1 : Abs
  Compare To Zero5 : simulink/Logic and Bit Operations/Compare To Zero  relop=<  OutDataTypeStr=boolean
  Integrator3 : Integrator
  Logical Operator3 : Logic  AllPortsSameDT=off  OutDataTypeStr=boolean
  Product3 : Product
  Vec2 : Gain  Gain=1.8
  Out4 (Energy losses) : Outport
  wires:
  Product3/1 -> Vec2/1
  current3/1 -> Abs1/1, Compare To Zero5/1
  Abs1/1 -> Product3/2
  Compare To Zero5/1 -> Logical Operator3/2
  Gate signal 3/1 -> Logical Operator3/1
  Vec2/1 -> Integrator3/1
  Integrator3/1 -> Out4 (Energy losses)/1
  Logical Operator3/1 -> Product3/1
